simulink model "transfer_function_1st_order_coefficient_input"  (R2013b)
settings: Solver=ode45  StartTime=0.0  StopTime=10.0  RelTol=1e-3
settings Model: Creator=Ahmed ElTahan  LastModifiedBy=MMSA
settings DataIOCC: SignalLoggingSaveFormat=ModelDataLogs
settings DebuggingCC: UnderspecifiedInitializationDetection=Simplified  MultiTaskDSMMsg=warning  MultiTaskCondExecSysMsg=none  StrictBusMsg=None
settings RTWCC: IncludeERTFirstTime=on
settings GRTTargetCC: CodeReplacementLibrary=None  CPPClassGenCompliant=on

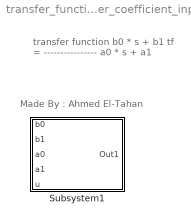
== system transfer_function_1st_order_coefficient_input ==
  note: Made By : Ahmed El-Tahan
  note: transfer function
      |       b0 * s + b1
      | tf = ----------------
      |       a0 * s + a1
  Subsystem1 : Subsystem

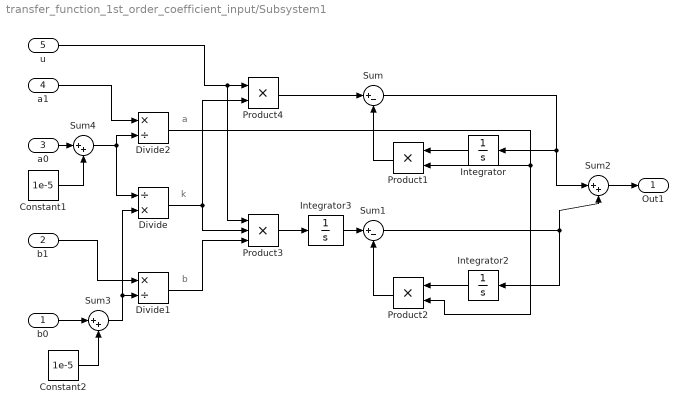
== system transfer_function_1st_order_coefficient_input/Subsystem1 ==
  note: b
  note: a
  note: k
  b0 : Inport
  b1 : Inport  Port=2
  a0 : Inport  Port=3
  a1 : Inport  Port=4
  u : Inport  Port=5
  Constant1 : Constant  Value=1e-5
  Constant2 : Constant  Value=1e-5
  Divide : Product  Inputs=/*
  Divide1 : Product  Inputs=*/
  Divide2 : Product  Inputs=*/
  Integrator : Integrator
  Integrator2 : Integrator
  Integrator3 : Integrator
  Product1 : Product
  Product2 : Product
  Product3 : Product  Inputs=3
  Product4 : Product
  Sum : Sum  Inputs=|+-
  Sum1 : Sum  Inputs=|+-
  Sum2 : Sum  Inputs=|++
  Sum3 : Sum  Inputs=|++
  Sum4 : Sum  Inputs=|++
  Out1 : Outport
  wires:
  Integrator/1 -> Product1/1
  Product1/1 -> Sum/2
  Sum/1 -> Sum2/1, Integrator/1
  Product4/1 -> Sum/1
  b1/1 -> Divide1/1
  a1/1 -> Divide2/1
  Divide2/1 -> Product2/2, Product1/2
  Divide1/1 -> Product3/3
  Integrator2/1 -> Product2/1
  Product2/1 -> Sum1/2
  Sum1/1 -> Sum2/2, Integrator2/1
  Integrator3/1 -> Sum1/1
  Product3/1 -> Integrator3/1
  Divide/1 -> Product4/2, Product3/2
  u/1 -> Product4/1, Product3/1
  Sum2/1 -> Out1/1
  Constant2/1 -> Sum3/2
  b0/1 -> Sum3/1
  Sum3/1 -> Divide/2, Divide1/2
  a0/1 -> Sum4/1
  Sum4/1 -> Divide2/2, Divide/1
  Constant1/1 -> Sum4/2
